simulink model "final_base_model"  (R2025b)
settings: Solver=VariableStepAuto  StartTime=0.0  StopTime=1000.0  RelTol=1e-3
libraries: nesl_utility x7, fl_lib x6, simulink x2

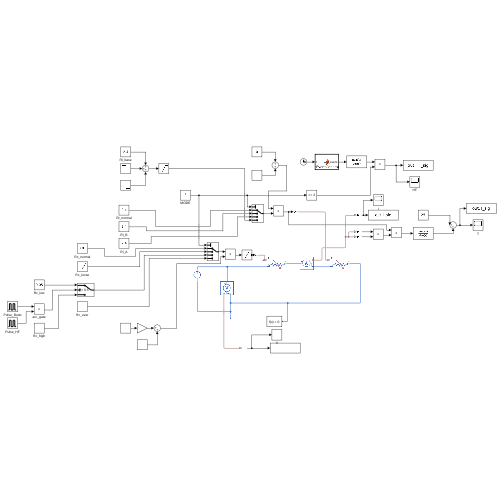
[thumbnail: Simulink's stored preview of the top-level diagram]
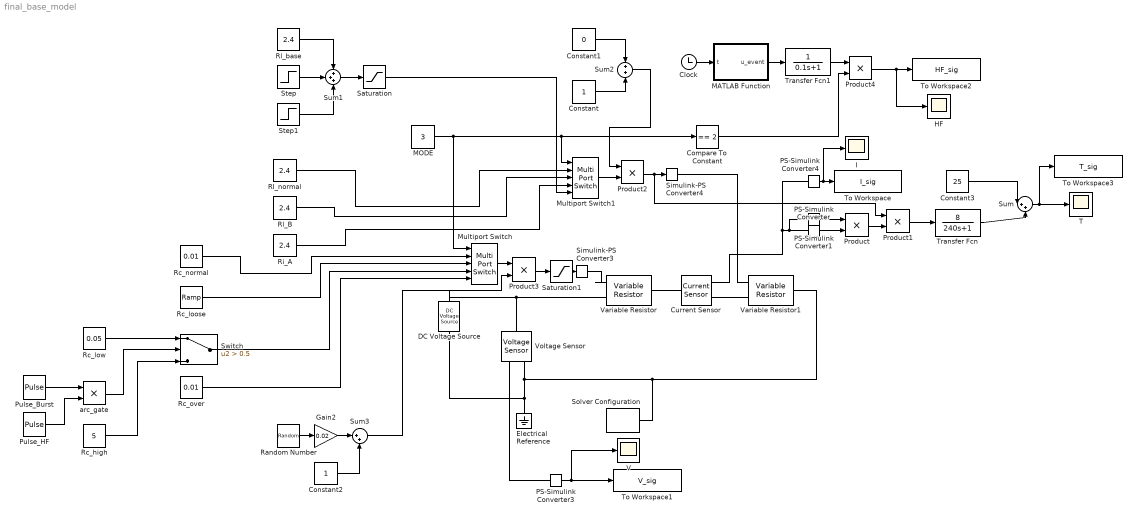
== system final_base_model ==
  Clock : Clock
  Compare To Constant : simulink/Logic and Bit Operations/Compare To Constant  relop===  const=2  OutDataTypeStr=boolean
  Constant : Constant
  Constant1 : Constant  Value=0
  Constant2 : Constant
  Constant3 : Constant  Value=25
  Current Sensor : fl_lib/Electrical/Electrical Sensors/Current Sensor
  DC Voltage Source : fl_lib/Electrical/Electrical Sources/DC Voltage Source  v0=24 V
  Electrical Reference : fl_lib/Electrical/Electrical Elements/Electrical Reference
  Gain2 : Gain  Gain=0.02
  HF : Scope
      settings: ActiveDisplayYMinimum=-0.011893117331512069  ActiveDisplayYMaximum=0.10703805598360866
  I : Scope
      settings: ActiveDisplayYMinimum=-0.081919423352700083  ActiveDisplayYMaximum=32.930912857738782  DataLoggingVariableName=ScopeData2
  MATLAB Function : MATLAB Function  TreatAsAtomicUnit=on  SystemSampleTime=0.01
  MODE : Constant  Value=3
  Multiport Switch : MultiPortSwitch  DataPortOrder=Zero-based contiguous  Inputs=4  zeroidx=on  SaturateOnIntegerOverflow=off  InputSameDT=off
  Multiport Switch1 : MultiPortSwitch  DataPortOrder=Zero-based contiguous  Inputs=4  zeroidx=on  SaturateOnIntegerOverflow=off  InputSameDT=off
  PS-Simulink Converter{,1,3..4} (4 alike) : nesl_utility/PS-Simulink Converter  PhysicalDomain=network_engine_domain  SubClassName=ps_output  LeftPortType=input  RightPortType=output  PseudoPeriodic=off  Frequencies=[]  VectorFormat=inherit  Unit=inherit  AffineConversion=off
  Product{,1..4} (5 alike) : Product
  Pulse_Burst : DiscretePulseGenerator  PulseType=Time based  Period=10  PulseWidth=5
  Pulse_HF : DiscretePulseGenerator  PulseType=Time based  Period=0.005  PulseWidth=30
  RI_normal : Constant  Value=2.4
  Random Number : RandomNumber  Variance=0.02  Seed=123  SampleTime=0.1
  Rc_high : Constant  Value=5
  Rc_loose : simulink/Sources/Ramp  slope=0.0002  start=0  InitialOutput=0.01
  Rc_low : Constant  Value=0.05
  Rc_normal : Constant  Value=0.01
  Rc_over : Constant  Value=0.01
  Ri_A : Constant  Value=2.4
  Rl_B : Constant  Value=2.4
  Rl_base : Constant  Value=2.4
  Saturation : Saturate  UpperLimit=10  LowerLimit=0.2
  Saturation1 : Saturate  UpperLimit=10  LowerLimit=1e-4
  Simulink-PS Converter3 : nesl_utility/Simulink-PS Converter  PhysicalDomain=network_engine_domain  SubClassName=ps_input  LeftPortType=input  RightPortType=output  PseudoPeriodic=off  Frequencies=[]  NoiseDistribution=none  NoiseParameters=[]  Unit=1  AffineConversion=off  FilteringAndDerivatives=provide  SimscapeFilterOrder=1  InputFilterTimeConstant=0.001  UdotUserProvided=0
  Simulink-PS Converter4 : nesl_utility/Simulink-PS Converter  PhysicalDomain=network_engine_domain  SubClassName=ps_input  LeftPortType=input  RightPortType=output  PseudoPeriodic=off  Frequencies=[]  NoiseDistribution=none  NoiseParameters=[]  Unit=1  AffineConversion=off  FilteringAndDerivatives=provide  SimscapeFilterOrder=1  InputFilterTimeConstant=0.001  UdotUserProvided=0
  Solver Configuration : nesl_utility/Solver Configuration  PhysicalDomain=network_engine_domain  SubClassName=solver  LeftPortType=input  RightPortType=generic  Tones=[]  Harmonics=[]  SimulateNoise=off  Profile=off  UseLocalSampling=off  EnableSwitchedLinearOptims=on  FrequencyDomain=off  UseCCode=off  RelTol=0.001  AbsTol=0.001  MinStep=1e-09  ToWorkspace=off  RevertToSquareIcSolve=off  NumHomotopyIterations=100  PhasorMode=off  PhasorModeNumHarmonics=1  ConsistencySolver=NEWTON_XTOL_AFTER_FTOL  IndexReductionMethod=DerivativeReplacement  DoDC=off  ResidualTolerance=1e-09  ConsistencyTolSource=GLOBAL  ConsistencyAbsTol=0.001  ConsistencyRelTol=0.001  ConsistencyTolFactor=0.001  UseLocalSolver=off  LocalSolverChoice=NE_BACKWARD_EULER_ADVANCER  ResolveIndetEquations=on  FunctionEvalNumThread=1  LocalSolverSampleTime=0.001  DoFixedCost=off  MaxNonlinIter=3  MaxModeIter=2  ComputeImpulses=off  ImpulseIterations=2  LinearAlgebra=auto  LinearAlgebraNumThread=0  EquationFormulation=NE_TIME_EF  DelaysMemoryBudget=1024  AutomaticFiltering=on  FilteringTimeConstant=0.001  PartitionStorageMethod=AS_NEEDED  PartitionMemoryBudget=1024  PartitionMethod=ROBUST  MultibodyUseLocalSolver=off  MultibodyLocalSolverChoice=ODE1  MultibodyLocalSolverSampleTime=0.001
  Step : Step  Time=3  After=-1.2  SampleTime=0
  Step1 : Step  Time=6  After=-0.4  SampleTime=0
  Sum : Sum  Inputs=|++
  Sum1 : Sum  Inputs=+++
  Sum2 : Sum
  Sum3 : Sum  Inputs=|++
  Switch : Switch  Criteria=u2 > Threshold  Threshold=0.5  SaturateOnIntegerOverflow=off  InputSameDT=off
  T : Scope
      settings: ActiveDisplayYMinimum=-666.28723161732682  ActiveDisplayYMaximum=6246.5850845559426
  To Workspace : ToWorkspace  VariableName=I_sig  SaveFormat=Timeseries  SampleTime=-1
  To Workspace1 : ToWorkspace  VariableName=V_sig  SaveFormat=Timeseries  SampleTime=-1
  To Workspace2 : ToWorkspace  VariableName=HF_sig  SaveFormat=Timeseries  SampleTime=-1
  To Workspace3 : ToWorkspace  VariableName=T_sig  SaveFormat=Timeseries  SampleTime=-1
  Transfer Fcn : TransferFcn  Numerator=[8]  Denominator=[240 1]
  Transfer Fcn1 : TransferFcn  Denominator=[0.1 1]
  V : Scope
      settings: ActiveDisplayYMinimum=14  ActiveDisplayYMaximum=34  DataLoggingVariableName=ScopeData3
  Variable Resistor : fl_lib/Electrical/Electrical Elements/Variable Resistor  Rmin=0.01 Ohm  thermalEnable=false  thermal_mass=1 J/K  i_specify=off  i_priority=None  i=0 A  i_nominal_specify=off  i_nominal_value=1  i_nominal_unit=A  v_specify=off  v_priority=None  v=0 V  v_nominal_specify=off  v_nominal_value=1  v_nominal_unit=V  T_specify=off  T_priority=None  T=300 K  T_nominal_specify=off  T_nominal_value=1  T_nominal_unit=K
  Variable Resistor1 : fl_lib/Electrical/Electrical Elements/Variable Resistor  Rmin=0.01 Ohm  thermalEnable=false  thermal_mass=1 J/K  i_specify=off  i_priority=None  i=0 A  i_nominal_specify=off  i_nominal_value=1  i_nominal_unit=A  v_specify=off  v_priority=None  v=0 V  v_nominal_specify=off  v_nominal_value=1  v_nominal_unit=V  T_specify=off  T_priority=None  T=300 K  T_nominal_specify=off  T_nominal_value=1  T_nominal_unit=K
  Voltage Sensor : fl_lib/Electrical/Electrical Sensors/Voltage Sensor
  arc_gate : Product
  wires:
  Constant3/1 -> Sum/1
  Transfer Fcn/1 -> Sum/2
  Product1/1 -> Transfer Fcn/1
  PS-Simulink Converter/1 -> Product/2
  PS-Simulink Converter1/1 -> Product/1
  Product/1 -> Product1/2
  Sum/1 -> T/1, To Workspace3/1
  Clock/1 -> MATLAB Function/1(t)
  MATLAB Function/1(u_event) -> Transfer Fcn1/1
  PS-Simulink Converter4/1 -> I/1, To Workspace/1
  PS-Simulink Converter3/1 -> V/1, To Workspace1/1
  Step/1 -> Sum1/2
  Step1/1 -> Sum1/3
  Rl_base/1 -> Sum1/1
  Sum1/1 -> Saturation/1
  RI_normal/1 -> Multiport Switch1/2
  Rl_B/1 -> Multiport Switch1/3
  Ri_A/1 -> Multiport Switch1/4
  Saturation/1 -> Multiport Switch1/5
  Rc_normal/1 -> Multiport Switch/2
  Rc_loose/1 -> Multiport Switch/3
  Rc_over/1 -> Multiport Switch/5
  Constant/1 -> Sum2/2
  Multiport Switch1/1 -> Product2/2
  Sum2/1 -> Product2/1
  Product2/1 -> Product1/1, Simulink-PS Converter4/1
  Pulse_HF/1 -> arc_gate/2
  Pulse_Burst/1 -> arc_gate/1
  Rc_low/1 -> Switch/1
  arc_gate/1 -> Switch/2
  Rc_high/1 -> Switch/3
  Switch/1 -> Multiport Switch/4
  Constant1/1 -> Sum2/1
  Random Number/1 -> Gain2/1
  Gain2/1 -> Sum3/1
  Constant2/1 -> Sum3/2
  Multiport Switch/1 -> Product3/1
  Sum3/1 -> Product3/2
  Product3/1 -> Saturation1/1
  Saturation1/1 -> Simulink-PS Converter3/1
  Transfer Fcn1/1 -> Product4/1
  Product4/1 -> HF/1, To Workspace2/1
  MODE/1 -> Multiport Switch/1, Compare To Constant/1, Multiport Switch1/1
  Compare To Constant/1 -> Product4/2
  connections:
  Current Sensor/LConn1 -- Variable Resistor/RConn1
  Current Sensor/RConn2 -- Variable Resistor1/LConn2
  Voltage Sensor/LConn1 -- DC Voltage Source/LConn1 -- Variable Resistor/LConn2
  Voltage Sensor/RConn2 -- Electrical Reference/LConn1 -- DC Voltage Source/RConn1 -- Solver Configuration/RConn1 -- Variable Resistor1/RConn1
  Current Sensor/RConn1 -- PS-Simulink Converter4/LConn1 -- PS-Simulink Converter1/LConn1 -- PS-Simulink Converter/LConn1
  PS-Simulink Converter3/LConn1 -- Voltage Sensor/RConn1
  Simulink-PS Converter4/RConn1 -- Variable Resistor1/LConn1
  Variable Resistor/LConn1 -- Simulink-PS Converter3/RConn1

== matlab function final_base_model/MATLAB Function ==
  data: t input; u_event output
function u_event = ArcEventGenerator(t)
persistent next_event initialized

if isempty(initialized)
    next_event = 10 + 20*rand(); % first event
    initialized = true;
end

u_event = 0;

if t >= next_event
    u_event = 1;
    next_event = t + (5 + 15*rand()); % next event after 5~20 s
end
